simulink model "FO_CTDNN_P_Bia_Para_2_V2"  (R2021b)
settings: Solver=ode5  StartTime=0.0  StopTime=40  FixedStep=0.005  RelTol=1e-3
(part 2 of 2)

== matlab function FO_CTDNN_P_Bia_Para_2_V2/Controller and Plant 4/Finite-time observer/Multi-layer neural network/J_i Update ==
  data: x_i_tilde input; J_dot output; W_hat input; J_hat input; x_bar input
function J_dot = J_update(x_i_tilde, W_hat, J_hat, x_bar)


eta_3 = 0.1;
eta_4 = 0.06;
% eta_5 = 0.1;

n_1 = 5;

alpha = tanh(J_hat' * x_bar);

% J_dot = eta_3 * sign(x_bar) * ( e_xi' * W_hat' * (eye(n_1) - diag(alpha.^2)) ) - eta_4 * norm(e_xi) * J_hat - eta_5  * J_hat; 

J_dot = eta_3 * sign(x_bar)/norm(sign(x_bar)) * ( x_i_tilde' * W_hat' * (eye(n_1) - diag(alpha.^2)) ) - eta_4 * norm(x_i_tilde) * J_hat; 

% J_dot = eta_3 * sign(x_bar) * ( e_xi' * W_hat' * (eye(n_1) - diag(alpha.^2)) ) - eta_4  * J_hat; 

end

== matlab function FO_CTDNN_P_Bia_Para_2_V2/Controller and Plant 4/Finite-time observer/Multi-layer neural network/Second layer ==
  data: W_hat input; E_hat output; mu input
function E_hat = second_layer(W_hat, mu)

%% From hidden layer to output layer
% w_hat = W_hat * mu(J_hat * x_i)


E_hat = W_hat' * mu; 

end

== matlab function FO_CTDNN_P_Bia_Para_2_V2/Controller and Plant 4/Finite-time observer/Multi-layer neural network/W_i Initialization ==
  data: W_0 output
function W_0 = W_ini()

n_1 = 5;
dimension = 3;

W_0 = 0.05*zeros(n_1,dimension);
% W_0 =randn(n, n_1);

end

== matlab function FO_CTDNN_P_Bia_Para_2_V2/Self Error Calculation 4/error_calculation ==
  data: v_di output; ref input; delta_x4 output; x_i input
function [v_di, delta_x4] = error_cal(ref, x_i)

%% Basic parameters

dimension = 3;
num_agent = 6;
serial_num = 4;

x_d = ref(1+dimension*0:dimension*num_agent);
v_d = ref(1+dimension*num_agent:2*dimension*num_agent);

x_di = x_d( (serial_num - 1)*dimension+1 : serial_num*dimension );
v_di = v_d( (serial_num - 1)*dimension+1 : serial_num*dimension );



delta_x4 = x_i - x_di;


end

== matlab function FO_CTDNN_P_Bia_Para_2_V2/Self Error Calculation 1/error_calculation ==
  data: v_di output; ref input; delta_x1 output; x_i input
function [v_di, delta_x1] = error_cal(ref, x_i)

%% Basic parameters

dimension = 3;
num_agent = 6;
serial_num = 1;

x_d = ref(1+dimension*0:dimension*num_agent);
v_d = ref(1+dimension*num_agent:2*dimension*num_agent);

x_di = x_d( (serial_num - 1)*dimension+1 : serial_num*dimension );
v_di = v_d( (serial_num - 1)*dimension+1 : serial_num*dimension );



delta_x1 = x_i - x_di;


end

== matlab function FO_CTDNN_P_Bia_Para_2_V2/Controller and Plant 4/Finite-time observer/Multi-layer neural network/W_i Update ==
  data: x_i_tilde input; W_dot output; W_hat input; mu input
function W_dot = W_update(x_i_tilde, W_hat, mu)


eta_1 = 15;
eta_2 = 0.1;
% eta_3 = 0.05;



% W_dot = eta_1 * mu * e_xi' - eta_2* norm(e_xi) * W_hat - eta_3 * W_hat; 

W_dot = eta_1 * mu * x_i_tilde' - eta_2* norm(x_i_tilde) * W_hat; 

% W_dot = eta_1 * mu * e_xi' - eta_2 * W_hat; 

end

== matlab function FO_CTDNN_P_Bia_Para_2_V2/Controller and Plant 4/Plant ==
  data: x_dot output; E_i output; x_i input; u_i input; t input
function [x_dot, E_i ] = model( x_i, u_i, t)

%% First-order plants for robots

Radius=[0.24;0.23;0.30;0.28;0.25;0.32];
Radius_esti=[0.21;0.25;0.33;0.24;0.28;0.29];

serial_num = 4;
dimension = 3; 

R = Radius(serial_num);
R_hat = Radius_esti(serial_num);

x = x_i(1);
y = x_i(2);
theta = x_i(3);

w_i =  [0.02 * cos(0.5* t+ pi/2) + 0.03 * exp( -abs(x) - 1 ) ; 0.03 * sin(0.2*t) + 0.02*tanh(y); 0.04*sin(0.1*t + theta) + 0.01 *tanh(theta)] ;
%d =  0.4* cos(0.5* t+ pi/2);


g_i = [-sin(theta) -sin(pi/3 - theta) sin(pi/3 + theta);
        cos(theta) -cos(pi/3 - theta) -cos(pi/3+ theta);
        1/R 1/R 1/R];
    
g_i_hat = [-sin(theta) -sin(pi/3 - theta) sin(pi/3 + theta);
        cos(theta) -cos(pi/3 - theta) -cos(pi/3+ theta);
        1/R_hat 1/R_hat 1/R_hat];
    
x_dot = g_i * u_i + w_i;


E_i = w_i + (g_i - g_i_hat) * u_i;




end

== matlab function FO_CTDNN_P_Bia_Para_2_V2/Controller and Plant 4/Smooth Projection ==
  data: u_i input; u_i output
function u_i = fcn(u_i)

tau_i = 0.24;
psi = 0.01;

dimension = 3;

for i = 1 : dimension
   if abs(u_i(i)) <= tau_i
       continue;
   else
       u_i(i) = sign(u_i(i)) * (tau_i + psi*exp((tau_i - abs(u_i(i)))/psi ));
   end 
end



end

== matlab function FO_CTDNN_P_Bia_Para_2_V2/Controller and Plant 4/controller ==
  data: v_di input; e_xi input; u_mi output; w_hat input; x_i input
function u_mi  = controller(v_di, e_xi, w_hat, x_i)


%% basic data
Radius_esti=[0.21;0.25;0.33;0.24;0.28;0.29];

serial_num = 4;
dimension = 3; 

R_hat=Radius_esti(serial_num);

theta = x_i(dimension);
k_p = 3;

g_i_hat = [-sin(theta) -sin(pi/3 - theta) sin(pi/3 + theta);
            cos(theta) -cos(pi/3 - theta) -cos(pi/3+ theta);
            1/R_hat 1/R_hat 1/R_hat];
    
%% First, we apply the smooth projection for uncertainty estimation
psi = 0.01;
w_m = 0.10;

for i = 1 : dimension
   if abs(w_hat(i)) <= w_m - psi
       continue;
   else
       w_hat(i) = sign(w_hat(i)) * (w_m - psi*exp( (w_m - psi - abs(w_hat(i)))/psi ));
   end 
end

%% Afterwards, we apply the smooth projection for formation maintain control input

% tau_i = 0.25;

u_mi = (g_i_hat)^(-1) * (- w_hat + v_di - k_p * e_xi);

% for i = 1 : dimension
%    if abs(u_mi(i)) <= tau_i
%        continue;
%    else
%        u_mi(i) = sign(u_mi(i)) * (tau_i + psi*exp((tau_i - abs(u_mi(i)))/psi ));
%    end 
% end


% u_i = - k_p * (g_i_hat)^(-1) * e_xi + u_mi; 




end

== matlab function FO_CTDNN_P_Bia_Para_2_V2/Controller and Plant 5/Local Error Calculate ==
  data: delta_x input; e_xi output; L input
function e_xi = local_error(delta_x, L)

%% Calculate the local formation tracking error from communication

dimension = 3;
serial_num = 5;

L_i = kron(L(serial_num, :) , eye(dimension));

e_xi = L_i * delta_x;







end

== matlab function FO_CTDNN_P_Bia_Para_2_V2/Controller and Plant 5/Finite-time observer/Multi-layer neural network/First layer ==
  data: J_hat input; mu output; x_bar input
function mu = first_layer(J_hat, x_bar)

%% From input layer to hidden layer
% mu = tanh(J_hat * x_i)

mu = tanh(J_hat' * x_bar);

end

== matlab function FO_CTDNN_P_Bia_Para_2_V2/Controller and Plant 5/Finite-time observer/Multi-layer neural network/J_i Initialization ==
  data: J_0 output
function J_0 = J_ini()

n_1 = 5;
dimension = 3;

J_0 = rand(2*dimension,n_1);

end

== matlab function FO_CTDNN_P_Bia_Para_2_V2/Controller and Plant 5/Finite-time observer/Multi-layer neural network/J_i Update ==
  data: x_i_tilde input; J_dot output; W_hat input; J_hat input; x_bar input
function J_dot = J_update(x_i_tilde, W_hat, J_hat, x_bar)


eta_3 = 0.1;
eta_4 = 0.06;
% eta_5 = 0.1;

n_1 = 5;

alpha = tanh(J_hat' * x_bar);

% J_dot = eta_3 * sign(x_bar) * ( e_xi' * W_hat' * (eye(n_1) - diag(alpha.^2)) ) - eta_4 * norm(e_xi) * J_hat - eta_5  * J_hat; 

J_dot = eta_3 * sign(x_bar)/norm(sign(x_bar)) * ( x_i_tilde' * W_hat' * (eye(n_1) - diag(alpha.^2)) ) - eta_4 * norm(x_i_tilde) * J_hat; 

% J_dot = eta_3 * sign(x_bar) * ( e_xi' * W_hat' * (eye(n_1) - diag(alpha.^2)) ) - eta_4  * J_hat; 

end

== matlab function FO_CTDNN_P_Bia_Para_2_V2/Controller and Plant 5/Finite-time observer/Multi-layer neural network/Second layer ==
  data: W_hat input; E_hat output; mu input
function E_hat = second_layer(W_hat, mu)

%% From hidden layer to output layer
% w_hat = W_hat * mu(J_hat * x_i)


E_hat = W_hat' * mu; 

end

== matlab function FO_CTDNN_P_Bia_Para_2_V2/Self Error Calculation 5/error_calculation ==
  data: v_di output; ref input; delta_x5 output; x_i input
function [v_di, delta_x5] = error_cal(ref, x_i)

%% Basic parameters

dimension = 3;
num_agent = 6;
serial_num = 5;

x_d = ref(1+dimension*0:dimension*num_agent);
v_d = ref(1+dimension*num_agent:2*dimension*num_agent);

x_di = x_d( (serial_num - 1)*dimension+1 : serial_num*dimension );
v_di = v_d( (serial_num - 1)*dimension+1 : serial_num*dimension );



delta_x5 = x_i - x_di;


end

== matlab function FO_CTDNN_P_Bia_Para_2_V2/Reference generator/reference ==
  data: t input; xd output
function xd = x_d(t)

% bias_x=0.2*t;
% bias_y=sin(0.3*t);

bias_x=2*cos(-0.15*t+pi) - 1;
bias_y=2*sin(-0.15*t+pi);

radius=2;
w=0;

phase=0;

x1=[radius*cos(w*t+pi/3*1+phase)+bias_x ; radius*sin(w*t+pi/3*1+phase)+bias_y ; 0];
x2=[radius*cos(w*t+pi/3*2+phase)+bias_x ; radius*sin(w*t+pi/3*2+phase)+bias_y ; 0];
x3=[radius*cos(w*t+pi/3*3+phase)+bias_x ; radius*sin(w*t+pi/3*3+phase)+bias_y ; 0];
x4=[radius*cos(w*t+pi/3*4+phase)+bias_x ; radius*sin(w*t+pi/3*4+phase)+bias_y ; 0];
x5=[radius*cos(w*t+pi/3*5+phase)+bias_x ; radius*sin(w*t+pi/3*5+phase)+bias_y ; 0];
x6=[radius*cos(w*t+pi/3*6+phase)+bias_x ; radius*sin(w*t+pi/3*6+phase)+bias_y ; 0];

xd=[x1;x2;x3;x4;x5;x6];

end

== matlab function FO_CTDNN_P_Bia_Para_2_V2/Controller and Plant 5/Finite-time observer/Multi-layer neural network/W_i Initialization ==
  data: W_0 output
function W_0 = W_ini()

n_1 = 5;
dimension = 3;

W_0 = 0.05*zeros(n_1,dimension);
% W_0 =randn(n, n_1);

end

== matlab function FO_CTDNN_P_Bia_Para_2_V2/Controller and Plant 5/Finite-time observer/Multi-layer neural network/W_i Update ==
  data: x_i_tilde input; W_dot output; W_hat input; mu input
function W_dot = W_update(x_i_tilde, W_hat, mu)


eta_1 = 15;
eta_2 = 0.1;
% eta_3 = 0.05;



% W_dot = eta_1 * mu * e_xi' - eta_2* norm(e_xi) * W_hat - eta_3 * W_hat; 

W_dot = eta_1 * mu * x_i_tilde' - eta_2* norm(x_i_tilde) * W_hat; 

% W_dot = eta_1 * mu * e_xi' - eta_2 * W_hat; 

end

== matlab function FO_CTDNN_P_Bia_Para_2_V2/Controller and Plant 5/Plant ==
  data: x_dot output; E_i output; x_i input; u_i input; t input
function [x_dot, E_i ] = model( x_i, u_i, t)

%% First-order plants for robots

Radius=[0.24;0.23;0.30;0.28;0.25;0.32];
Radius_esti=[0.21;0.25;0.33;0.24;0.28;0.29];


serial_num = 5;
dimension = 3; 

R = Radius(serial_num);
R_hat = Radius_esti(serial_num);

x = x_i(1);
y = x_i(2);
theta = x_i(3);

w_i =  [0.02 * cos(0.5* t+ pi/2) + 0.03 * exp( -abs(x) - 1 ) ; 0.03 * sin(0.2*t) + 0.02*tanh(y); 0.04*sin(0.1*t + theta) + 0.01 *tanh(theta)] ;
%d =  0.4* cos(0.5* t+ pi/2);


g_i = [-sin(theta) -sin(pi/3 - theta) sin(pi/3 + theta);
        cos(theta) -cos(pi/3 - theta) -cos(pi/3+ theta);
        1/R 1/R 1/R];
    
g_i_hat = [-sin(theta) -sin(pi/3 - theta) sin(pi/3 + theta);
        cos(theta) -cos(pi/3 - theta) -cos(pi/3+ theta);
        1/R_hat 1/R_hat 1/R_hat];
    
x_dot = g_i * u_i + w_i;


E_i = w_i + (g_i - g_i_hat) * u_i;




end

== matlab function FO_CTDNN_P_Bia_Para_2_V2/Controller and Plant 5/Smooth Projection ==
  data: u_i input; u_i output
function u_i = fcn(u_i)

tau_i = 0.24;
psi = 0.01;

dimension = 3;

for i = 1 : dimension
   if abs(u_i(i)) <= tau_i
       continue;
   else
       u_i(i) = sign(u_i(i)) * (tau_i + psi*exp((tau_i - abs(u_i(i)))/psi ));
   end 
end



end

== matlab function FO_CTDNN_P_Bia_Para_2_V2/Controller and Plant 5/controller ==
  data: v_di input; e_xi input; u_mi output; w_hat input; x_i input
function u_mi  = controller(v_di, e_xi, w_hat, x_i)


%% basic data
Radius_esti=[0.21;0.25;0.33;0.24;0.28;0.29];

serial_num = 5;
dimension = 3; 

R_hat=Radius_esti(serial_num);

theta = x_i(dimension);
k_p = 3;

g_i_hat = [-sin(theta) -sin(pi/3 - theta) sin(pi/3 + theta);
            cos(theta) -cos(pi/3 - theta) -cos(pi/3+ theta);
            1/R_hat 1/R_hat 1/R_hat];
    
%% First, we apply the smooth projection for uncertainty estimation
psi = 0.01;
w_m = 0.10;

for i = 1 : dimension
   if abs(w_hat(i)) <= w_m - psi
       continue;
   else
       w_hat(i) = sign(w_hat(i)) * (w_m - psi*exp( (w_m - psi - abs(w_hat(i)))/psi ));
   end 
end

%% Afterwards, we apply the smooth projection for formation maintain control input

% tau_i = 0.25;

u_mi = (g_i_hat)^(-1) * (- w_hat + v_di - k_p * e_xi);

% for i = 1 : dimension
%    if abs(u_mi(i)) <= tau_i
%        continue;
%    else
%        u_mi(i) = sign(u_mi(i)) * (tau_i + psi*exp((tau_i - abs(u_mi(i)))/psi ));
%    end 
% end


% u_i = - k_p * (g_i_hat)^(-1) * e_xi + u_mi; 




end

== matlab function FO_CTDNN_P_Bia_Para_2_V2/Controller and Plant 6/Local Error Calculate ==
  data: delta_x input; e_xi output; L input
function e_xi = local_error(delta_x, L)

%% Calculate the local formation tracking error from communication

dimension = 3;
serial_num = 6;

L_i = kron(L(serial_num, :) , eye(dimension));

e_xi = L_i * delta_x;







end

== matlab function FO_CTDNN_P_Bia_Para_2_V2/Controller and Plant 6/Finite-time observer/Multi-layer neural network/First layer ==
  data: J_hat input; mu output; x_bar input
function mu = first_layer(J_hat, x_bar)

%% From input layer to hidden layer
% mu = tanh(J_hat * x_i)

mu = tanh(J_hat' * x_bar);

end

== matlab function FO_CTDNN_P_Bia_Para_2_V2/Controller and Plant 6/Finite-time observer/Multi-layer neural network/J_i Initialization ==
  data: J_0 output
function J_0 = J_ini()

n_1 = 5;
dimension = 3;

J_0 = rand(2*dimension,n_1);

end

== matlab function FO_CTDNN_P_Bia_Para_2_V2/Controller and Plant 6/Finite-time observer/Multi-layer neural network/J_i Update ==
  data: x_i_tilde input; J_dot output; W_hat input; J_hat input; x_bar input
function J_dot = J_update(x_i_tilde, W_hat, J_hat, x_bar)


eta_3 = 0.1;
eta_4 = 0.06;
% eta_5 = 0.1;

n_1 = 5;

alpha = tanh(J_hat' * x_bar);

% J_dot = eta_3 * sign(x_bar) * ( e_xi' * W_hat' * (eye(n_1) - diag(alpha.^2)) ) - eta_4 * norm(e_xi) * J_hat - eta_5  * J_hat; 

J_dot = eta_3 * sign(x_bar)/norm(sign(x_bar)) * ( x_i_tilde' * W_hat' * (eye(n_1) - diag(alpha.^2)) ) - eta_4 * norm(x_i_tilde) * J_hat; 

% J_dot = eta_3 * sign(x_bar) * ( e_xi' * W_hat' * (eye(n_1) - diag(alpha.^2)) ) - eta_4  * J_hat; 

end

== matlab function FO_CTDNN_P_Bia_Para_2_V2/Reference generator/reference1 ==
  data: t input; vd output
function vd = v_d(t)



% v1=[0.2 ; 0.3*cos(0.3*t) ; 0];
% v2=[0.2 ; 0.3*cos(0.3*t) ; 0];
% v3=[0.2 ; 0.3*cos(0.3*t) ; 0];
% v4=[0.2 ; 0.3*cos(0.3*t) ; 0];
% v5=[0.2 ; 0.3*cos(0.3*t) ; 0];
% v6=[0.2 ; 0.3*cos(0.3*t) ; 0];



v1=[0.3 *sin(-0.15*t+pi) ; - 0.3 *cos(-0.15*t+pi) ; 0];
v2=[0.3 *sin(-0.15*t+pi) ; - 0.3 *cos(-0.15*t+pi) ; 0];
v3=[0.3 *sin(-0.15*t+pi) ; - 0.3 *cos(-0.15*t+pi) ; 0];
v4=[0.3 *sin(-0.15*t+pi) ; - 0.3 *cos(-0.15*t+pi) ; 0];
v5=[0.3 *sin(-0.15*t+pi) ; - 0.3 *cos(-0.15*t+pi) ; 0];
v6=[0.3 *sin(-0.15*t+pi) ; - 0.3 *cos(-0.15*t+pi) ; 0];

vd=[v1;v2;v3;v4;v5;v6];

end

== matlab function FO_CTDNN_P_Bia_Para_2_V2/Self Error Calculation 6/error_calculation ==
  data: v_di output; ref input; delta_x6 output; x_i input
function [v_di, delta_x6] = error_cal(ref, x_i)

%% Basic parameters

dimension = 3;
num_agent = 6;
serial_num = 6;

x_d = ref(1+dimension*0:dimension*num_agent);
v_d = ref(1+dimension*num_agent:2*dimension*num_agent);

x_di = x_d( (serial_num - 1)*dimension+1 : serial_num*dimension );
v_di = v_d( (serial_num - 1)*dimension+1 : serial_num*dimension );



delta_x6 = x_i - x_di;


end

== matlab function FO_CTDNN_P_Bia_Para_2_V2/Controller and Plant 6/Finite-time observer/Multi-layer neural network/Second layer ==
  data: W_hat input; E_hat output; mu input
function E_hat = second_layer(W_hat, mu)

%% From hidden layer to output layer
% w_hat = W_hat * mu(J_hat * x_i)


E_hat = W_hat' * mu; 

end

== matlab function FO_CTDNN_P_Bia_Para_2_V2/Controller and Plant 6/Finite-time observer/Multi-layer neural network/W_i Initialization ==
  data: W_0 output
function W_0 = W_ini()

n_1 = 5;
dimension = 3;

W_0 = 0.05*zeros(n_1,dimension);
% W_0 =randn(n, n_1);

end

== matlab function FO_CTDNN_P_Bia_Para_2_V2/Controller and Plant 6/Finite-time observer/Multi-layer neural network/W_i Update ==
  data: x_i_tilde input; W_dot output; W_hat input; mu input
function W_dot = W_update(x_i_tilde, W_hat, mu)


eta_1 = 15;
eta_2 = 0.1;
% eta_3 = 0.05;



% W_dot = eta_1 * mu * e_xi' - eta_2* norm(e_xi) * W_hat - eta_3 * W_hat; 

W_dot = eta_1 * mu * x_i_tilde' - eta_2* norm(x_i_tilde) * W_hat; 

% W_dot = eta_1 * mu * e_xi' - eta_2 * W_hat; 

end

== matlab function FO_CTDNN_P_Bia_Para_2_V2/Controller and Plant 6/Plant ==
  data: x_dot output; E_i output; x_i input; u_i input; t input
function [x_dot, E_i ] = model( x_i, u_i, t)

%% First-order plants for robots

Radius=[0.24;0.23;0.30;0.28;0.25;0.32];
Radius_esti=[0.21;0.25;0.33;0.24;0.28;0.29];


serial_num = 6;
dimension = 3; 

R = Radius(serial_num);
R_hat = Radius_esti(serial_num);

x = x_i(1);
y = x_i(2);
theta = x_i(3);

w_i =  [0.02 * cos(0.5* t+ pi/2) + 0.03 * exp( -abs(x) - 1 ) ; 0.03 * sin(0.2*t) + 0.02*tanh(y); 0.04*sin(0.1*t + theta) + 0.01 *tanh(theta)] ;
%d =  0.4* cos(0.5* t+ pi/2);


g_i = [-sin(theta) -sin(pi/3 - theta) sin(pi/3 + theta);
        cos(theta) -cos(pi/3 - theta) -cos(pi/3+ theta);
        1/R 1/R 1/R];
    
g_i_hat = [-sin(theta) -sin(pi/3 - theta) sin(pi/3 + theta);
        cos(theta) -cos(pi/3 - theta) -cos(pi/3+ theta);
        1/R_hat 1/R_hat 1/R_hat];
    
x_dot = g_i * u_i + w_i;


E_i = w_i + (g_i - g_i_hat) * u_i;




end

== matlab function FO_CTDNN_P_Bia_Para_2_V2/Controller and Plant 6/Smooth Projection ==
  data: u_i input; u_i output
function u_i = fcn(u_i)

tau_i = 0.24;
psi = 0.01;

dimension = 3;

for i = 1 : dimension
   if abs(u_i(i)) <= tau_i
       continue;
   else
       u_i(i) = sign(u_i(i)) * (tau_i + psi*exp((tau_i - abs(u_i(i)))/psi ));
   end 
end



end

== matlab function FO_CTDNN_P_Bia_Para_2_V2/Controller and Plant 6/controller ==
  data: v_di input; e_xi input; u_mi output; w_hat input; x_i input
function u_mi  = controller(v_di, e_xi, w_hat, x_i)


%% basic data
Radius_esti=[0.21;0.25;0.33;0.24;0.28;0.29];

serial_num = 6;
dimension = 3; 

R_hat=Radius_esti(serial_num);

theta = x_i(dimension);
k_p = 3;

g_i_hat = [-sin(theta) -sin(pi/3 - theta) sin(pi/3 + theta);
            cos(theta) -cos(pi/3 - theta) -cos(pi/3+ theta);
            1/R_hat 1/R_hat 1/R_hat];
    
%% First, we apply the smooth projection for uncertainty estimation
psi = 0.01;
w_m = 0.10;

for i = 1 : dimension
   if abs(w_hat(i)) <= w_m - psi
       continue;
   else
       w_hat(i) = sign(w_hat(i)) * (w_m - psi*exp( (w_m - psi - abs(w_hat(i)))/psi ));
   end 
end

%% Afterwards, we apply the smooth projection for formation maintain control input

% tau_i = 0.25;

u_mi = (g_i_hat)^(-1) * (- w_hat + v_di - k_p * e_xi);

% for i = 1 : dimension
%    if abs(u_mi(i)) <= tau_i
%        continue;
%    else
%        u_mi(i) = sign(u_mi(i)) * (tau_i + psi*exp((tau_i - abs(u_mi(i)))/psi ));
%    end 
% end


% u_i = - k_p * (g_i_hat)^(-1) * e_xi + u_mi; 




end

== matlab function FO_CTDNN_P_Bia_Para_2_V2/Controller and Plant 1/Finite-time observer/Observer ==
  data: x_i_hat input; x_i input; u_i input; x_hat_dot output; E_hat input; x_i_tilde output
function [x_hat_dot, x_i_tilde] = observer(x_i_hat, x_i, u_i, E_hat)

%% observer itself
Radius_esti=[0.21;0.25;0.33;0.24;0.28;0.29];

serial_num = 1;
dimension = 3; 

gamma_i = diag([12,12,18]);

beta_i = 0.9;

R_hat=Radius_esti(serial_num);

theta = x_i(dimension);
    
g_i_hat = [-sin(theta) -sin(pi/3 - theta) sin(pi/3 + theta);
            cos(theta) -cos(pi/3 - theta) -cos(pi/3+ theta);
            1/R_hat 1/R_hat 1/R_hat];

x_i_tilde = x_i - x_i_hat;

x_hat_dot = g_i_hat * u_i + E_hat + gamma_i * diag( abs(x_i_tilde).^(beta_i - 1) ) * x_i_tilde;


end

== matlab function FO_CTDNN_P_Bia_Para_2_V2/Controller and Plant 1/Finite-time observer/Multi-layer neural network/J_i Initialization ==
  data: J_0 output
function J_0 = J_ini()

n_1 = 5;
dimension = 3;

J_0 = rand(2*dimension,n_1);

end

== matlab function FO_CTDNN_P_Bia_Para_2_V2/Controller and Plant 2/Finite-time observer/Observer ==
  data: x_i_hat input; x_i input; u_i input; x_hat_dot output; E_hat input; x_i_tilde output
function [x_hat_dot, x_i_tilde] = observer(x_i_hat, x_i, u_i, E_hat)

%% observer itself
Radius_esti=[0.21;0.25;0.33;0.24;0.28;0.29];

serial_num = 2;
dimension = 3; 

gamma_i = diag([12,12,18]);

beta_i = 0.9;

R_hat=Radius_esti(serial_num);

theta = x_i(dimension);
    
g_i_hat = [-sin(theta) -sin(pi/3 - theta) sin(pi/3 + theta);
            cos(theta) -cos(pi/3 - theta) -cos(pi/3+ theta);
            1/R_hat 1/R_hat 1/R_hat];

x_i_tilde = x_i - x_i_hat;

x_hat_dot = g_i_hat * u_i + E_hat + gamma_i * diag( abs(x_i_tilde).^(beta_i - 1) ) * x_i_tilde;


end

== matlab function FO_CTDNN_P_Bia_Para_2_V2/Controller and Plant 3/Finite-time observer/Observer ==
  data: x_i_hat input; x_i input; u_i input; x_hat_dot output; E_hat input; x_i_tilde output
function [x_hat_dot, x_i_tilde] = observer(x_i_hat, x_i, u_i, E_hat)

%% observer itself
Radius_esti=[0.21;0.25;0.33;0.24;0.28;0.29];

serial_num = 3;
dimension = 3; 

gamma_i = diag([12,12,18]);

beta_i = 0.9;

R_hat=Radius_esti(serial_num);

theta = x_i(dimension);
    
g_i_hat = [-sin(theta) -sin(pi/3 - theta) sin(pi/3 + theta);
            cos(theta) -cos(pi/3 - theta) -cos(pi/3+ theta);
            1/R_hat 1/R_hat 1/R_hat];

x_i_tilde = x_i - x_i_hat;

x_hat_dot = g_i_hat * u_i + E_hat + gamma_i * diag( abs(x_i_tilde).^(beta_i - 1) ) * x_i_tilde;


end

== matlab function FO_CTDNN_P_Bia_Para_2_V2/Controller and Plant 4/Finite-time observer/Observer ==
  data: x_i_hat input; x_i input; u_i input; x_hat_dot output; E_hat input; x_i_tilde output
function [x_hat_dot, x_i_tilde] = observer(x_i_hat, x_i, u_i, E_hat)

%% observer itself
Radius_esti=[0.21;0.25;0.33;0.24;0.28;0.29];

serial_num = 4;
dimension = 3; 

gamma_i = diag([12,12,18]);

beta_i = 0.9;

R_hat=Radius_esti(serial_num);

theta = x_i(dimension);
    
g_i_hat = [-sin(theta) -sin(pi/3 - theta) sin(pi/3 + theta);
            cos(theta) -cos(pi/3 - theta) -cos(pi/3+ theta);
            1/R_hat 1/R_hat 1/R_hat];

x_i_tilde = x_i - x_i_hat;

x_hat_dot = g_i_hat * u_i + E_hat + gamma_i * diag( abs(x_i_tilde).^(beta_i - 1) ) * x_i_tilde;


end

== matlab function FO_CTDNN_P_Bia_Para_2_V2/Controller and Plant 5/Finite-time observer/Observer ==
  data: x_i_hat input; x_i input; u_i input; x_hat_dot output; E_hat input; x_i_tilde output
function [x_hat_dot, x_i_tilde] = observer(x_i_hat, x_i, u_i, E_hat)

%% observer itself
Radius_esti=[0.21;0.25;0.33;0.24;0.28;0.29];

serial_num = 5;
dimension = 3; 

gamma_i = diag([12,12,18]);

beta_i = 0.9;

R_hat=Radius_esti(serial_num);

theta = x_i(dimension);
    
g_i_hat = [-sin(theta) -sin(pi/3 - theta) sin(pi/3 + theta);
            cos(theta) -cos(pi/3 - theta) -cos(pi/3+ theta);
            1/R_hat 1/R_hat 1/R_hat];

x_i_tilde = x_i - x_i_hat;

x_hat_dot = g_i_hat * u_i + E_hat + gamma_i * diag( abs(x_i_tilde).^(beta_i - 1) ) * x_i_tilde;


end

== matlab function FO_CTDNN_P_Bia_Para_2_V2/Controller and Plant 6/Finite-time observer/Observer ==
  data: x_i_hat input; x_i input; u_i input; x_hat_dot output; E_hat input; x_i_tilde output
function [x_hat_dot, x_i_tilde] = observer(x_i_hat, x_i, u_i, E_hat)

%% observer itself
Radius_esti=[0.21;0.25;0.33;0.24;0.28;0.29];

serial_num = 6;
dimension = 3; 

gamma_i = diag([12,12,18]);

beta_i = 0.9;

R_hat=Radius_esti(serial_num);

theta = x_i(dimension);
    
g_i_hat = [-sin(theta) -sin(pi/3 - theta) sin(pi/3 + theta);
            cos(theta) -cos(pi/3 - theta) -cos(pi/3+ theta);
            1/R_hat 1/R_hat 1/R_hat];

x_i_tilde = x_i - x_i_hat;

x_hat_dot = g_i_hat * u_i + E_hat + gamma_i * diag( abs(x_i_tilde).^(beta_i - 1) ) * x_i_tilde;


end

== matlab function FO_CTDNN_P_Bia_Para_2_V2/Controller and Plant 1/Finite-time observer/Multi-layer neural network/W_i Initialization ==
  data: W_0 output
function W_0 = W_ini()

n_1 = 5;
dimension = 3;

W_0 = 0.05*zeros(n_1,dimension);
% W_0 =randn(n, n_1);

end

== matlab function FO_CTDNN_P_Bia_Para_2_V2/Controller and Plant 1/U_abs ==
  data: u_i input; u_int output
function  u_int = fcn(u_i)

u_ab = abs(u_i);

u_int = u_ab(1) + u_ab(2) + u_ab(3);


end

== matlab function FO_CTDNN_P_Bia_Para_2_V2/Controller and Plant 2/U_abs ==
  data: u_i input; u_int output
function  u_int = fcn(u_i)

u_ab = abs(u_i);

u_int = u_ab(1) + u_ab(2) + u_ab(3);


end

== matlab function FO_CTDNN_P_Bia_Para_2_V2/Controller and Plant 3/U_abs ==
  data: u_i input; u_int output
function  u_int = fcn(u_i)

u_ab = abs(u_i);

u_int = u_ab(1) + u_ab(2) + u_ab(3);


end

== matlab function FO_CTDNN_P_Bia_Para_2_V2/Controller and Plant 4/U_abs ==
  data: u_i input; u_int output
function  u_int = fcn(u_i)

u_ab = abs(u_i);

u_int = u_ab(1) + u_ab(2) + u_ab(3);


end

== matlab function FO_CTDNN_P_Bia_Para_2_V2/Controller and Plant 5/U_abs ==
  data: u_i input; u_int output
function  u_int = fcn(u_i)

u_ab = abs(u_i);

u_int = u_ab(1) + u_ab(2) + u_ab(3);


end

== matlab function FO_CTDNN_P_Bia_Para_2_V2/Controller and Plant 6/U_abs ==
  data: u_i input; u_int output
function  u_int = fcn(u_i)

u_ab = abs(u_i);

u_int = u_ab(1) + u_ab(2) + u_ab(3);


end

== matlab function FO_CTDNN_P_Bia_Para_2_V2/Controller and Plant 1/Finite-time observer/Multi-layer neural network/J_i Update ==
  data: x_i_tilde input; J_dot output; W_hat input; J_hat input; x_bar input
function J_dot = J_update(x_i_tilde, W_hat, J_hat, x_bar)


eta_3 = 0.1;
eta_4 = 0.06;
% eta_5 = 0.1;

n_1 = 5;

alpha = tanh(J_hat' * x_bar);

% J_dot = eta_3 * sign(x_bar) * ( e_xi' * W_hat' * (eye(n_1) - diag(alpha.^2)) ) - eta_4 * norm(e_xi) * J_hat - eta_5  * J_hat; 

J_dot = eta_3 * sign(x_bar)/norm(sign(x_bar)) * ( x_i_tilde' * W_hat' * (eye(n_1) - diag(alpha.^2)) ) - eta_4 * norm(x_i_tilde) * J_hat; 

% J_dot = eta_3 * sign(x_bar) * ( e_xi' * W_hat' * (eye(n_1) - diag(alpha.^2)) ) - eta_4  * J_hat; 

end

== matlab function FO_CTDNN_P_Bia_Para_2_V2/Controller and Plant 1/Finite-time observer/Multi-layer neural network/W_i Update ==
  data: x_i_tilde input; W_dot output; W_hat input; mu input
function W_dot = W_update(x_i_tilde, W_hat, mu)


eta_1 = 15;
eta_2 = 0.1;
% eta_3 = 0.05;



% W_dot = eta_1 * mu * e_xi' - eta_2* norm(e_xi) * W_hat - eta_3 * W_hat; 

W_dot = eta_1 * mu * x_i_tilde' - eta_2* norm(x_i_tilde) * W_hat; 

% W_dot = eta_1 * mu * e_xi' - eta_2 * W_hat; 

end

== matlab function FO_CTDNN_P_Bia_Para_2_V2/Controller and Plant 1/Finite-time observer/Multi-layer neural network/First layer ==
  data: J_hat input; mu output; x_bar input
function mu = first_layer(J_hat, x_bar)

%% From input layer to hidden layer
% mu = tanh(J_hat * x_i)

mu = tanh(J_hat' * x_bar);

end

== matlab function FO_CTDNN_P_Bia_Para_2_V2/Controller and Plant 1/Finite-time observer/Multi-layer neural network/Second layer ==
  data: W_hat input; E_hat output; mu input
function E_hat = second_layer(W_hat, mu)

%% From hidden layer to output layer
% w_hat = W_hat * mu(J_hat * x_i)


E_hat = W_hat' * mu; 

end
